simulink model "FDIBenchMark_BLW_Part2"  (Simulink 7.0)
settings: Solver=ode45  StartTime=0.0  StopTime=4400  FixedStep=Ts  RelTol=1e-12
InitFcn:
  | FDIBenchMarkData
undefined symbols (not defined in the file or in its folder): a, Addt, Addt2, alpha, alpha_gc, Apb, Apb1, Apb2, Bddt, Bddt2, Bpb, Bpb1, Bpb2, Cddt, Constant_Beta_1_m1, Constant_Beta_3_m1, Constant_Omega_r_m1, Constant_tau_gc, Cpb, Cpb1, Cpb2, Cq, eta_gc, Gain_Beta_2_m2, Gain_Omega_r_m2, H, k, L, m, m_vw, omega_n, P_r, R, r, r0, rho, seed, T_sample, Ts, turb_int, turbulence_seeds, u0, xi
libraries: simulink x13
(part 2 of 2)

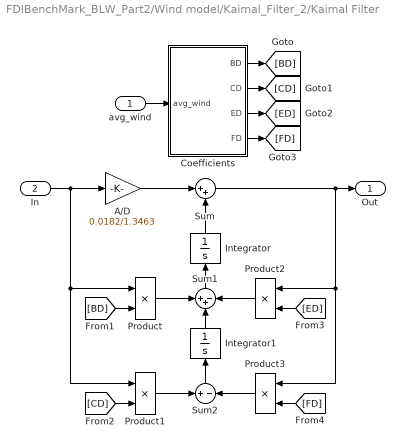
== system FDIBenchMark_BLW_Part2/Wind model/Kaimal_Filter_2/Kaimal Filter ==
  avg_wind : Inport  OutDataType=sfix(16)  OutScaling=2^0
  In : Inport  Port=2  OutDataType=sfix(16)  OutScaling=2^0
  A/D : Gain  Gain=0.0182/1.3463  ParameterDataType=sfix(16)  ParameterScaling=2^0  OutDataType=sfix(16)  OutScaling=2^0  SaturateOnIntegerOverflow=on
  Coefficients : Subsystem
  Integrator : Integrator  Orientation=up
  Integrator1 : Integrator  Orientation=up
  Product : Product  OutDataType=sfix(16)  OutScaling=2^0  SaturateOnIntegerOverflow=on
  Product1 : Product  OutDataType=sfix(16)  OutScaling=2^0  SaturateOnIntegerOverflow=on
  Product2 : Product  Orientation=left  OutDataType=sfix(16)  OutScaling=2^0  SaturateOnIntegerOverflow=on
  Product3 : Product  Orientation=left  OutDataType=sfix(16)  OutScaling=2^0  SaturateOnIntegerOverflow=on
  Sum : Sum  Inputs=|++  OutDataType=sfix(16)  OutScaling=2^0  SaturateOnIntegerOverflow=on
  Sum1 : Sum  Orientation=up  Inputs=++-  OutDataType=sfix(16)  OutScaling=2^0  SaturateOnIntegerOverflow=on
  Sum2 : Sum  Orientation=up  Inputs=+|-  OutDataType=sfix(16)  OutScaling=2^0  SaturateOnIntegerOverflow=on
  Out : Outport  OutDataType=sfix(16)  OutScaling=2^0
  wires:
  A/D/1 -> Sum/1
  Integrator/1 -> Sum/2
  Sum1/1 -> Integrator/1
  Product/1 -> Sum1/1
  Integrator1/1 -> Sum1/2
  Product2/1 -> Sum1/3
  Sum2/1 -> Integrator1/1
  Product3/1 -> Sum2/2
  Product1/1 -> Sum2/1
  Sum/1 -> Product2/1, Product3/1, Out/1
  In/1 -> A/D/1, Product/1, Product1/1
  [BD] -> Product/2
  [CD] -> Product1/2
  [ED] -> Product2/2
  [FD] -> Product3/2
  Coefficients/1(BD) -> [BD]
  Coefficients/2(CD) -> [CD]
  Coefficients/3(ED) -> [ED]
  Coefficients/4(FD) -> [FD]
  avg_wind/1 -> Coefficients/1(avg_wind)

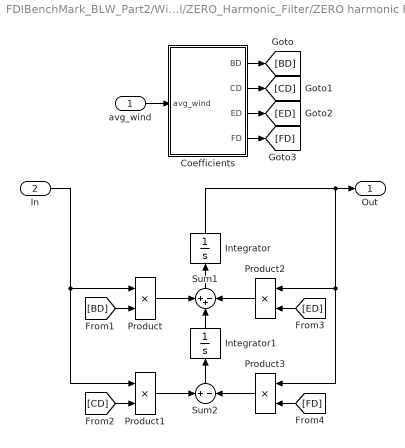
== system FDIBenchMark_BLW_Part2/Wind model/ZERO_Harmonic_Filter/ZERO harmonic Filter ==
  avg_wind : Inport  OutDataType=sfix(16)  OutScaling=2^0
  In : Inport  Port=2  OutDataType=sfix(16)  OutScaling=2^0
  Coefficients : Subsystem
  Integrator : Integrator  Orientation=up
  Integrator1 : Integrator  Orientation=up
  Product : Product  OutDataType=sfix(16)  OutScaling=2^0  SaturateOnIntegerOverflow=on
  Product1 : Product  OutDataType=sfix(16)  OutScaling=2^0  SaturateOnIntegerOverflow=on
  Product2 : Product  Orientation=left  OutDataType=sfix(16)  OutScaling=2^0  SaturateOnIntegerOverflow=on
  Product3 : Product  Orientation=left  OutDataType=sfix(16)  OutScaling=2^0  SaturateOnIntegerOverflow=on
  Sum1 : Sum  Orientation=up  Inputs=++-  OutDataType=sfix(16)  OutScaling=2^0  SaturateOnIntegerOverflow=on
  Sum2 : Sum  Orientation=up  Inputs=+|-  OutDataType=sfix(16)  OutScaling=2^0  SaturateOnIntegerOverflow=on
  Out : Outport  OutDataType=sfix(16)  OutScaling=2^0
  wires:
  Integrator/1 -> Product2/1, Product3/1, Out/1
  Sum1/1 -> Integrator/1
  Product/1 -> Sum1/1
  Integrator1/1 -> Sum1/2
  Product2/1 -> Sum1/3
  Sum2/1 -> Integrator1/1
  Product3/1 -> Sum2/2
  Product1/1 -> Sum2/1
  In/1 -> Product/1, Product1/1
  [BD] -> Product/2
  [CD] -> Product1/2
  [ED] -> Product2/2
  [FD] -> Product3/2
  Coefficients/1(BD) -> [BD]
  Coefficients/2(CD) -> [CD]
  Coefficients/3(ED) -> [ED]
  Coefficients/4(FD) -> [FD]
  avg_wind/1 -> Coefficients/1(avg_wind)

== system FDIBenchMark_BLW_Part2/Wind model/3rd_Harmonic_Filter1/3rd harmonic Filter/Coefficients ==
  avg_wind : Inport  OutDataType=sfix(16)  OutScaling=2^0
  BD coeff : Fcn  Expr=0.2766/0.3691/(r/u(1))
  CD coeff : Fcn  Expr=0.0307/0.3691/(r/u(1))^2
  ED coeff : Fcn  Expr=1.7722/0.3691/(r/u(1))
  FD coeff : Fcn  Expr=1/0.3691/(r/u(1))^2
  BD : Outport  OutDataType=sfix(16)  OutScaling=2^0
  CD : Outport  Port=2  OutDataType=sfix(16)  OutScaling=2^0
  ED : Outport  Port=3  OutDataType=sfix(16)  OutScaling=2^0
  FD : Outport  Port=4  OutDataType=sfix(16)  OutScaling=2^0
  wires:
  FD coeff/1 -> FD/1
  ED coeff/1 -> ED/1
  CD coeff/1 -> CD/1
  BD coeff/1 -> BD/1
  avg_wind/1 -> FD coeff/1, ED coeff/1, CD coeff/1, BD coeff/1

== system FDIBenchMark_BLW_Part2/Wind model/Kaimal_Filter_1/Kaimal Filter/Coefficients ==
  avg_wind : Inport  OutDataType=sfix(16)  OutScaling=2^0
  BD coeff : Fcn  Expr=1.3653/1.3463/(L/2/pi/u(1))
  CD coeff : Fcn  Expr=0.9846/1.3463/(L/2/pi/u(1))^2
  ED coeff : Fcn  Expr=3.7593/1.3463/(L/2/pi/u(1))
  FD coeff : Fcn  Expr=1/1.3463/(L/2/pi/u(1))^2
  BD : Outport  OutDataType=sfix(16)  OutScaling=2^0
  CD : Outport  Port=2  OutDataType=sfix(16)  OutScaling=2^0
  ED : Outport  Port=3  OutDataType=sfix(16)  OutScaling=2^0
  FD : Outport  Port=4  OutDataType=sfix(16)  OutScaling=2^0
  wires:
  FD coeff/1 -> FD/1
  ED coeff/1 -> ED/1
  CD coeff/1 -> CD/1
  BD coeff/1 -> BD/1
  avg_wind/1 -> FD coeff/1, ED coeff/1, CD coeff/1, BD coeff/1

== system FDIBenchMark_BLW_Part2/Wind model/Kaimal_Filter_2/Kaimal Filter/Coefficients ==
  avg_wind : Inport  OutDataType=sfix(16)  OutScaling=2^0
  BD coeff : Fcn  Expr=1.3653/1.3463/(L/2/pi/u(1))
  CD coeff : Fcn  Expr=0.9846/1.3463/(L/2/pi/u(1))^2
  ED coeff : Fcn  Expr=3.7593/1.3463/(L/2/pi/u(1))
  FD coeff : Fcn  Expr=1/1.3463/(L/2/pi/u(1))^2
  BD : Outport  OutDataType=sfix(16)  OutScaling=2^0
  CD : Outport  Port=2  OutDataType=sfix(16)  OutScaling=2^0
  ED : Outport  Port=3  OutDataType=sfix(16)  OutScaling=2^0
  FD : Outport  Port=4  OutDataType=sfix(16)  OutScaling=2^0
  wires:
  avg_wind/1 -> BD coeff/1, CD coeff/1, ED coeff/1, FD coeff/1
  BD coeff/1 -> BD/1
  CD coeff/1 -> CD/1
  ED coeff/1 -> ED/1
  FD coeff/1 -> FD/1

== system FDIBenchMark_BLW_Part2/Wind model/ZERO_Harmonic_Filter/ZERO harmonic Filter/Coefficients ==
  avg_wind : Inport  OutDataType=sfix(16)  OutScaling=2^0
  BD coeff : Fcn  Expr=4.7869/7.6823/(r/u(1))
  CD coeff : Fcn  Expr=0.9904/7.6823/(r/u(1))^2
  ED coeff : Fcn  Expr=7.3518/7.6823/(r/u(1))
  FD coeff : Fcn  Expr=1/7.6823/(r/u(1))^2
  BD : Outport  OutDataType=sfix(16)  OutScaling=2^0
  CD : Outport  Port=2  OutDataType=sfix(16)  OutScaling=2^0
  ED : Outport  Port=3  OutDataType=sfix(16)  OutScaling=2^0
  FD : Outport  Port=4  OutDataType=sfix(16)  OutScaling=2^0
  wires:
  avg_wind/1 -> BD coeff/1, CD coeff/1, ED coeff/1, FD coeff/1
  BD coeff/1 -> BD/1
  CD coeff/1 -> CD/1
  ED coeff/1 -> ED/1
  FD coeff/1 -> FD/1
